simulink model "Discrete_Time_Integrator_extX0_verif"  (Simulink 7.2)
settings: Solver=ode45  StartTime=0.0  StopTime=10.0  RelTol=1e-3
undefined symbols (not defined in the file): integrator_sample
settings Model: Creator=Romain  LastModifiedBy=Romain
settings OptimizationCC: ExpressionDepthLimit=128
settings DebuggingCC: SolverPrmCheckMsg=none  FcnCallInpInsideContextMsg=Enable All  StateNameClashWarn=none  StrictBusMsg=ErrorLevel1
settings CodeAppCC: CustomSymbolStrType=$N$R$M_T
settings GRTTargetCC: TargetFunctionLibrary=C89/C90 (ANSI)

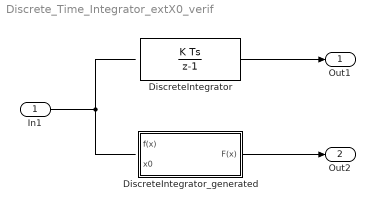
== system Discrete_Time_Integrator_extX0_verif ==
  In1 : Inport  OutDataTypeStr=double  DataType=double
  DiscreteIntegrator : DiscreteIntegrator  InitialConditionSource=external  InitialConditionMode=State only (most efficient)
  DiscreteIntegrator_generated : Subsystem  TreatAsAtomicUnit=on
  Out1 : Outport
  Out2 : Outport  Port=2
  wires:
  In1/1 -> ?
  DiscreteIntegrator/1 -> Out1/1
  DiscreteIntegrator_generated/1(F(x)) -> Out2/1

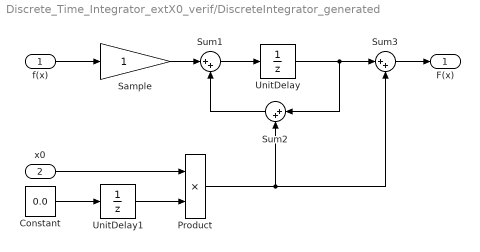
== system Discrete_Time_Integrator_extX0_verif/DiscreteIntegrator_generated ==
  f(x) : Inport
  x0 : Inport  Port=2
  Constant : Constant  Value=0.0  SampleTime=integrator_sample
  Product : Product  RndMeth=Zero
  Sample : Gain
  Sum1 : Sum  RequirementInfo={} %GIDa_8424ec66_cd37_4ff3_a9a4_e973dbf558d7  Inputs=|++
  Sum2 : Sum  RequirementInfo={} %GIDa_f121c1c8_ced0_4403_ae01_4e16f836dc82  Orientation=left  Inputs=|++
  Sum3 : Sum  RequirementInfo={} %GIDa_294813f4_d3f8_4461_a0e1_46b737124caa  Inputs=|++
  UnitDelay : UnitDelay
  UnitDelay1 : UnitDelay  X0=1
  F(x) : Outport  RequirementInfo={} %GIDa_466fe182_920e_40cf_8814_67447caa0806
  wires:
  Sum1/1 -> UnitDelay/1
  Sample/1 -> Sum1/1
  UnitDelay/1 -> Sum3/1, Sum2/1
  Sum2/1 -> Sum1/2
  Product/1 -> Sum3/2, Sum2/2
  UnitDelay1/1 -> Product/2
  Constant/1 -> UnitDelay1/1
  f(x)/1 -> Sample/1
  x0/1 -> Product/1
  Sum3/1 -> F(x)/1
